simulink model "A3P2"  (R2023b)
settings: Solver=VariableStepAuto  StartTime=0.0  StopTime=0.2  MaxStep=0.001  RelTol=1e-3
settings Model: Creator=amandeepbehera  LastModifiedBy=amandeepbehera

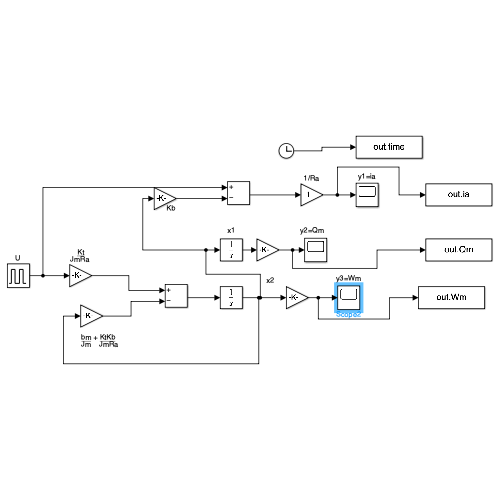
[thumbnail: Simulink's stored preview of the top-level diagram]
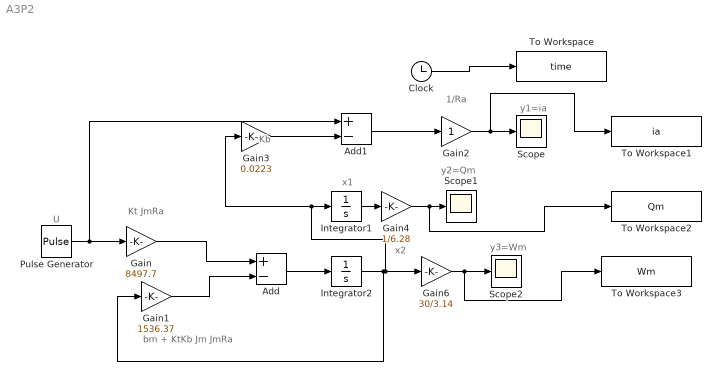
== system A3P2 ==
  note: y1=ia
  note: Kb
  note: 1/Ra
  note: bm + KtKb
      | Jm JmRa
  note: Kt
      | JmRa
  note: y2=Qm
  note: y3=Wm
  note: x1
  note: U
  note: x2
  Add : Sum  Inputs=+-
  Add1 : Sum  Inputs=+-
  Clock : Clock
  Gain : Gain  Gain=8497.7
  Gain1 : Gain  Gain=1536.37
  Gain2 : Gain
  Gain3 : Gain  Gain=0.0223
  Gain4 : Gain  Gain=1/6.28
  Gain6 : Gain  Gain=30/3.14
  Integrator1 : Integrator
  Integrator2 : Integrator
  Pulse Generator : DiscretePulseGenerator  PulseType=Time based  Amplitude=10  Period=.2  PulseWidth=50
  Scope : Scope
  Scope1 : Scope
  Scope2 : Scope
  To Workspace : ToWorkspace  VariableName=time  SaveFormat=Timeseries  SampleTime=-1
  To Workspace1 : ToWorkspace  VariableName=ia  SaveFormat=Timeseries  SampleTime=-1
  To Workspace2 : ToWorkspace  VariableName=Qm  SaveFormat=Timeseries  SampleTime=-1
  To Workspace3 : ToWorkspace  VariableName=Wm  SaveFormat=Timeseries  SampleTime=-1
  wires:
  Gain6/1 -> To Workspace3/1, Scope2/1
  Integrator2/1 -> Gain1/1, Gain6/1, Gain3/1, Integrator1/1
  Add/1 -> Integrator2/1
  Gain1/1 -> Add/2
  Gain/1 -> Add/1
  Pulse Generator/1 -> Add1/1, Gain/1
  Gain2/1 -> To Workspace1/1, Scope/1
  Add1/1 -> Gain2/1
  Gain3/1 -> Add1/2
  Clock/1 -> To Workspace/1
  Gain4/1 -> Scope1/1, To Workspace2/1
  Integrator1/1 -> Gain4/1
